simulink model "Motor_Control_Test"  (R2017b)
settings: Solver=VariableStepAuto  StartTime=0.0  StopTime=10.0  RelTol=1e-3
undefined symbols (not defined in the file): IC, quadModel
libraries: NLGCToolbox x1, simulink x1
settings Model: Creator=hoang  LastModifiedBy=hoang

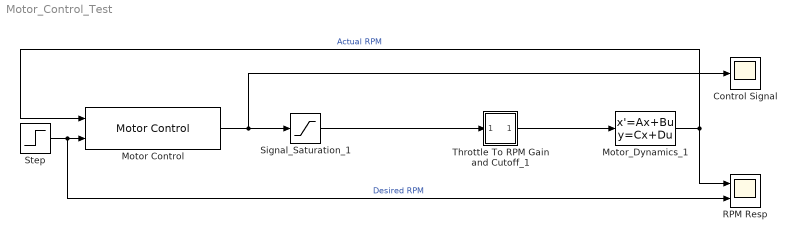
== system Motor_Control_Test ==
  Control Signal : Scope
  Motor Control : NLGCToolbox/Motor Control  k=6  Km=quadModel.cr  Ts=1/60  T=quadModel.T  Rdt=100  Rdx=2  b=quadModel.b
      settings: SourceProductName=Thinh - NLGC for Quadrotor
  Motor_Dynamics_1 : StateSpace  A=-1/quadModel.T  C=1/quadModel.T  D=0  InitialCondition=IC.w1*quadModel.T
  RPM Resp : Scope  NumInputPorts=2
  Signal_Saturation_1 : Saturate  UpperLimit=100  LowerLimit=0
  Step : Step  Time=0  After=0  SampleTime=0
  Throttle To RPM Gain and Cutoff_1 : Subsystem
  wires:
  Throttle To RPM Gain and Cutoff_1/1(Out5) -> Motor_Dynamics_1/1
  Signal_Saturation_1/1 -> Throttle To RPM Gain and Cutoff_1/1(In5)
  Motor Control/1 -> Control Signal/1, Signal_Saturation_1/1
  Motor_Dynamics_1/1 -> RPM Resp/1, Motor Control/1  "Actual RPM"
  Step/1 -> RPM Resp/2, Motor Control/2  "Desired RPM"

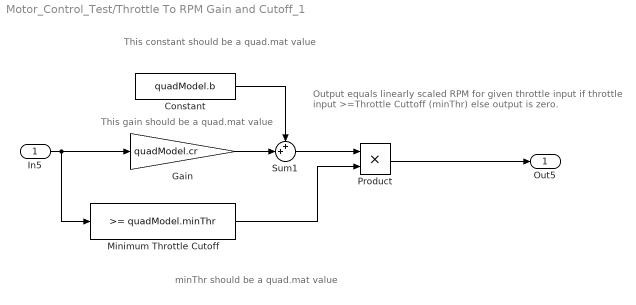
== system Motor_Control_Test/Throttle To RPM Gain and Cutoff_1 ==
  note: minThr should be a quad.mat value
  note: This gain should be a quad.mat value
  note: This constant should be a quad.mat value
  note: Output equals linearly scaled RPM
      | for given throttle input if throttle input >=Throttle Cuttoff (minThr)
      | else output is zero.
  In5 : Inport
  Constant : Constant  Value=quadModel.b
  Gain : Gain  Gain=quadModel.cr
  Minimum Throttle Cutoff : simulink/Logic and Bit Operations/Compare To Constant  relop=>=  const=quadModel.minThr  OutDataTypeStr=uint8
  Product : Product
  Sum1 : Sum  Inputs=++|
  Out5 : Outport
  wires:
  Minimum Throttle Cutoff/1 -> Product/2
  Product/1 -> Out5/1
  In5/1 -> Gain/1, Minimum Throttle Cutoff/1
  Gain/1 -> Sum1/2
  Sum1/1 -> Product/1
  Constant/1 -> Sum1/1
